simulink model "PIL_NO_RPI"  (R2021a)
settings: Solver=FixedStepAuto  StartTime=0.0  StopTime=50  FixedStep=0.001  RelTol=1e-3  EnableMultiTasking=on
undefined symbols (not defined in the file or in its folder): act_dmp, act_omega, Actuator, Aerodynamics, aMode, Autopilot, c_b_WGS, c_be, c_flat, c_grav, c_h_geop0, c_h_geope, c_pa0, c_pe, c_r0, c_rot, c_rsma, c_Tmp0, d_siB_0, d_siB_max, d_siB_min, dd_siB_max, dd_siB_min, DiscIntNeverNeededParam, e_pa, e_Tmp, fin_maxrate, flag_I_act_switch, flag_I_aero_switch, flag_I_flat, flag_I_gravity_switch, flag_I_rot, hcr, HIL_Data, JMMM_0, JMMM_e, JSPB_e, lat_0, lon_0, Mass_Props, mB_0, mM_0, mM_e, p, pBII_0, phi, pMPB, pNPB, propellant_kg, prp_FBPB, prp_mdot, prp_T, psi, pSPB, q, qEG_0, qIB_0, qIE_0, r, sgc ... (+28)
libraries: simulink x46, simulink_extras x10, aerolibcommonsys x4
(part 17 of 21)

== system PIL_NO_RPI/Non-linear Flight Dynamic Model1/Subsystem1/GRM_Airframe/rb_eom/calc_bus_flight_dyn_bus_entries/q12_from_T12/q_R^3(R) ==
  DCM : Inport
  q_R^3(R) = TRUE : EnablePort
  (1-r11-r22+r33)^1/2 : Sqrt  SaturateOnIntegerOverflow=on
  Add : Sum  Inputs=+--+
  Constant : Constant
  Divide : Product  Inputs=*/
  Divide1 : Product  Inputs=*/
  Divide2 : Product  Inputs=*/
  Gain : Gain  Gain=0.5
  Saturation : Saturate  UpperLimit=inf  LowerLimit=eps
      settings: AttributesFormatString=|
      | %<UpperLimit>
      | %<LowerLimit>
  Subtract : Sum
  Subtract1 : Sum  Inputs=+-
  Subtract2 : Sum
  Vector Concatenate : Concatenate  NumInputs=4
  dcm11 : Selector  NumberOfDimensions=2  IndexMode=Zero-based  InputPortWidth=3  IndexOptions=Index vector (dialog),Index vector (dialog)  Indices=0,0  OutputSizes=1,1
  dcm12 : Selector  NumberOfDimensions=2  IndexMode=Zero-based  InputPortWidth=3  IndexOptions=Index vector (dialog),Index vector (dialog)  Indices=0,1  OutputSizes=1,1
  dcm13 : Selector  NumberOfDimensions=2  IndexMode=Zero-based  InputPortWidth=3  IndexOptions=Index vector (dialog),Index vector (dialog)  Indices=0,2  OutputSizes=1,1
  dcm21 : Selector  NumberOfDimensions=2  IndexMode=Zero-based  InputPortWidth=3  IndexOptions=Index vector (dialog),Index vector (dialog)  Indices=1,0  OutputSizes=1,1
  dcm22 : Selector  NumberOfDimensions=2  IndexMode=Zero-based  InputPortWidth=3  IndexOptions=Index vector (dialog),Index vector (dialog)  Indices=1,1  OutputSizes=1,1
  dcm23 : Selector  NumberOfDimensions=2  IndexMode=Zero-based  InputPortWidth=3  IndexOptions=Index vector (dialog),Index vector (dialog)  Indices=1,2  OutputSizes=1,1
  dcm31 : Selector  NumberOfDimensions=2  IndexMode=Zero-based  InputPortWidth=3  IndexOptions=Index vector (dialog),Index vector (dialog)  Indices=2,0  OutputSizes=1,1
  dcm32 : Selector  NumberOfDimensions=2  IndexMode=Zero-based  InputPortWidth=3  IndexOptions=Index vector (dialog),Index vector (dialog)  Indices=2,1  OutputSizes=1,1
  dcm33 : Selector  NumberOfDimensions=2  IndexMode=Zero-based  InputPortWidth=3  IndexOptions=Index vector (dialog),Index vector (dialog)  Indices=2,2  OutputSizes=1,1
  q_R^3(R) : Outport  VectorParamsAs1DForOutWhenUnconnected=off
  wires:
  Saturation/1 -> Divide1/2, Divide2/2, Vector Concatenate/3, Divide/2  "q3"
  Gain/1 -> q_R^3(R)/1
  Divide/1 -> Vector Concatenate/4  "q4"
  Vector Concatenate/1 -> Gain/1
  (1-r11-r22+r33)^1/2/1 -> Saturation/1
  Divide2/1 -> Vector Concatenate/2  "q2"
  Divide1/1 -> Vector Concatenate/1  "q1"
  Subtract/1 -> Divide2/1  "dcm23+dcm32"
  Subtract2/1 -> Divide1/1  "dcm31+dcm13"
  Subtract1/1 -> Divide/1  "dcm12-dcm21"
  dcm12/1 -> Subtract1/1  "dcm12"
  dcm21/1 -> Subtract1/2  "dcm21"
  dcm13/1 -> Subtract2/2  "dcm13"
  dcm31/1 -> Subtract2/1  "dcm31"
  dcm32/1 -> Subtract/2  "dcm32"
  dcm23/1 -> Subtract/1  "dcm23"
  Add/1 -> (1-r11-r22+r33)^1/2/1
  dcm33/1 -> Add/4  "dcm33"
  dcm22/1 -> Add/3  "dcm22"
  dcm11/1 -> Add/2  "dcm11"
  Constant/1 -> Add/1
  DCM/1 -> dcm13/1, dcm31/1, dcm23/1, dcm32/1, dcm11/1, dcm22/1, dcm33/1, dcm21/1, dcm12/1

== system PIL_NO_RPI/Non-linear Flight Dynamic Model1/Subsystem1/GRM_Airframe/rb_eom/eom_6dof/Rigid_Body_EOM_6_DOF/Integration ==
  d_pBII : Inport
  d_vBII : Inport  Port=2
  d_qIB : Inport  Port=3
  d_wBIB : Inport  Port=4
  x0 : Inport  Port=5
  Bus Creator : BusCreator  Inputs=6
  Reshape : Reshape  OutputDimensionality=Customize  OutputDimensions=[13,1]
  Reshape1 : Reshape  OutputDimensionality=Customize  OutputDimensions=[3,1]
  Reshape2 : Reshape  OutputDimensionality=Customize  OutputDimensions=[3,1]
  Selector : Selector  IndexMode=Zero-based  InputPortWidth=13  IndexOptions=Index vector (dialog)  Indices=0:2  OutputSizes=3
  Selector1 : Selector  IndexMode=Zero-based  InputPortWidth=13  IndexOptions=Index vector (dialog)  Indices=3:5  OutputSizes=3
  Selector2 : Selector  IndexMode=Zero-based  InputPortWidth=13  IndexOptions=Index vector (dialog)  Indices=6:9  OutputSizes=3
  Selector3 : Selector  IndexMode=Zero-based  InputPortWidth=13  IndexOptions=Index vector (dialog)  Indices=10:12  OutputSizes=3
  Vector Concatenate : Concatenate  NumInputs=4  ConcatenateDimension=2
  integration_eom : Integrator  InitialConditionSource=external
  normalize_quaternion : Subsystem
      mask help: normalize a quaternion
      mask Help:
      | Name:
      | 
      |     normalize_quaternion
      | 
      | Description:
      | 
      |     This block normalizes the quaternion q21. It should be used as a
      |     safety measure when computing quaternions.
      | 
      | Inputs  [size] [data type] [unit]:
      | 
      |     attitude quaternion q21  [4] [double] [-]
      | 
      | Outputs  [size] [data type] [unit]:
      | 
      |     normalized attitude quaternion q21  [4] [double] [-]
      mask Display: disp (' norm(q)')
  eom : Outport  VectorParamsAs1DForOutWhenUnconnected=off
  wires:
  normalize_quaternion/1(q_normalized) -> Bus Creator/3  "qIB"
  Reshape2/1 -> Bus Creator/6  "d_vBII"
  Reshape1/1 -> Bus Creator/5  "d_wBIB"
  Reshape/1 -> integration_eom/1  "d_x"
  d_pBII/1 -> Vector Concatenate/1
  d_vBII/1 -> Vector Concatenate/2, Reshape2/1
  d_qIB/1 -> Vector Concatenate/3
  d_wBIB/1 -> Vector Concatenate/4, Reshape1/1
  Vector Concatenate/1 -> Reshape/1  "d_x"
  integration_eom/1 -> Selector2/1, Selector3/1, Selector/1, Selector1/1  "x"
  x0/1 -> integration_eom/2
  Selector/1 -> Bus Creator/1  "pBII"
  Selector1/1 -> Bus Creator/2  "vBII"
  Selector2/1 -> normalize_quaternion/1(q)  "qIB"
  Selector3/1 -> Bus Creator/4  "wBIB"
  Bus Creator/1 -> eom/1  "eom_bus"

== system PIL_NO_RPI/Non-linear Flight Dynamic Model1/Subsystem1/GRM_Airframe/rb_eom/eom_6dof/Rigid_Body_EOM_6_DOF/T12_from_q12 ==
  note: Inputs [size]:
      |
      | quaternion q12 [4]
  note: Outputs [size]:
      |
      | direction cosine matrix T12 [3x3]
  q12 : Inport  PortDimensions=4
  Add : Sum  Inputs=+--+
  Add1 : Sum  Inputs=+-
  Add2 : Sum  Inputs=+-
  Add3 : Sum  Inputs=+-
  Add4 : Sum
  Add5 : Sum
  Add6 : Sum  Inputs=-+-+
  Add7 : Sum  Inputs=--++
  Add8 : Sum
  Demux : Demux
  Gain{1..12} (12 alike) : Gain  Gain=2
  Math Function{,1..11} (12 alike) : Math  Operator=square  SignedPower=on  SaturateOnIntegerOverflow=on
  Product{,1..11} (12 alike) : Product
  Vector Concatenate : Concatenate  NumInputs=3
  Vector Concatenate1 : Concatenate  NumInputs=3
  Vector Concatenate2 : Concatenate  NumInputs=3
  Vector Concatenate3 : Concatenate  NumInputs=3  Mode=Multidimensional array  ConcatenateDimension=2
  T12 : Outport  PortDimensions=[3 3]  VectorParamsAs1DForOutWhenUnconnected=off
  wires:
  Product10/1 -> Gain11/1
  Product11/1 -> Gain12/1
  Gain11/1 -> Add8/1
  Gain12/1 -> Add8/2
  Math Function8/1 -> Add7/1
  Math Function9/1 -> Add7/2
  Math Function11/1 -> Add7/4
  Math Function10/1 -> Add7/3
  Math Function4/1 -> Add6/1
  Math Function5/1 -> Add6/2
  Math Function7/1 -> Add6/4
  Math Function6/1 -> Add6/3
  Product8/1 -> Gain9/1
  Product9/1 -> Gain10/1
  Gain9/1 -> Add5/1
  Gain10/1 -> Add5/2
  Product6/1 -> Gain7/1
  Product7/1 -> Gain8/1
  Gain7/1 -> Add4/1
  Gain8/1 -> Add4/2
  Product4/1 -> Gain5/1
  Product5/1 -> Gain6/1
  Gain5/1 -> Add3/1
  Gain6/1 -> Add3/2
  Product2/1 -> Gain3/1
  Product3/1 -> Gain4/1
  Gain3/1 -> Add2/1
  Gain4/1 -> Add2/2
  Gain2/1 -> Add1/2
  Gain1/1 -> Add1/1
  Product1/1 -> Gain2/1
  Product/1 -> Gain1/1
  Math Function3/1 -> Add/4
  Math Function2/1 -> Add/3
  Math Function1/1 -> Add/2
  Math Function/1 -> Add/1
  Add7/1 -> Vector Concatenate2/3  "dcm33"
  Add8/1 -> Vector Concatenate2/2  "dcm23"
  Add3/1 -> Vector Concatenate2/1  "dcm13"
  Add2/1 -> Vector Concatenate1/3  "dcm32"
  Add6/1 -> Vector Concatenate1/2  "dcm22"
  Add4/1 -> Vector Concatenate1/1  "dcm12"
  Add5/1 -> Vector Concatenate/3  "dcm31"
  Add1/1 -> Vector Concatenate/2  "dcm21"
  Add/1 -> Vector Concatenate/1  "dcm11"
  Vector Concatenate1/1 -> Vector Concatenate3/2
  Vector Concatenate2/1 -> Vector Concatenate3/3
  Vector Concatenate/1 -> Vector Concatenate3/1
  Vector Concatenate3/1 -> T12/1
  Demux/4 -> Product3/2, Product11/2, Math Function11/1, Product5/2, Math Function3/1, Product1/2, Product9/2, Product7/2, Math Function7/1  "q4 / q0"
  Demux/3 -> Math Function2/1, Product1/1, Product8/2, Product7/1, Math Function6/1, Product10/2, Math Function10/1, Product4/2, Product2/2  "q3"
  Demux/2 -> Math Function1/1, Product/2, Product9/1, Product6/2, Math Function5/1, Math Function9/1, Product10/1, Product5/1, Product2/1  "q2"
  Demux/1 -> Product6/1, Math Function4/1, Math Function8/1, Product11/1, Product4/1, Product3/1, Math Function/1, Product/1, Product8/1  "q1"
  q12/1 -> Demux/1

== system PIL_NO_RPI/Non-linear Flight Dynamic Model1/Subsystem1/GRM_Airframe/rb_eom/eom_6dof/Rigid_Body_EOM_6_DOF/rb_eom_6dof ==
  note: d_wBIB = JBB \ (MBTB - d_JBB * wBIB - wBIB x (JBB*wBIB))
  FBTB : Inport
  mB : Inport  Port=2
  JBB : Inport  Port=3
  MBTB : Inport  Port=4
  d_JBB : Inport  Port=5
  qIB : Inport  Port=6
  vBII : Inport  Port=7
  wBIB : Inport  Port=8
  Divide : Product  Inputs=*/
  Divide1 : Product  Inputs=/*  Multiplication=Matrix(*)
  Product : Product  Multiplication=Matrix(*)
  Product1 : Product  Multiplication=Matrix(*)
  Saturation : Saturate  UpperLimit=Inf  LowerLimit=1e-6
      settings: AttributesFormatString=|
      | %<UpperLimit>
      | %<LowerLimit>
  Subtract : Sum  Inputs=+--
  calc_d_qIB : Subsystem
  cross_product : Subsystem
      mask help: cross product r3 = r1 x r2
      mask Help:
      | Name:
      | 
      |     cross_product
      | 
      | Description:
      | 
      |     This block implements the cross product r3 = r1 x r2.
      | 
      | Inputs  [size] [data type] [unit]:
      | 
      |     vector 1  [3] [double] [-]
      |     vector 2  [3] [double] [-]
      | 
      | Outputs  [size] [data type] [unit]:
      | 
      |     resulting vector  [3] [double] [-]
      mask Display: disp(' r3 = r1 x r2')
  r2_from_r1_trans_q21 : Subsystem
      mask help: transforms a vector from frame 1 to frame 2 by a quaternion
      mask Help:
      | Name:
      | 
      |     r2_from_r1_trans_q21
      | 
      | Description:
      | 
      |     This block implements the transformation of a vector from the frame 1
      |     to the frame 2 using the appropriate quaternion.
      | 
      | Inputs  [size] [data type] [unit]:
      | 
      |     vector in frame 1  [3] [double] [-]
      |     attitude quaternion q21  [4] [double] [-]
      | 
      | Outputs  [size] [data type] [unit]:
      | 
      |     vector in frame 2  [3] [double] [-]
      mask Display:
      | port_label('input', 1, 'r1')
      | port_label('input', 2, 'q21')
      | port_label('output', 1, 'r2')
      | disp('r_2 = q_{21} {\bf\cdot} r_1 {\bf\cdot} q_{21}^{\bf\prime}','texmode','on')
  d_pBII : Outport  VectorParamsAs1DForOutWhenUnconnected=off
  d_vBII : Outport  Port=2  VectorParamsAs1DForOutWhenUnconnected=off
  d_qIB : Outport  Port=3  VectorParamsAs1DForOutWhenUnconnected=off
  d_wBIB : Outport  Port=4  VectorParamsAs1DForOutWhenUnconnected=off
  wires:
  Saturation/1 -> Divide/2
  calc_d_qIB/1(d_qIB) -> d_qIB/1
  MBTB/1 -> Subtract/1
  Subtract/1 -> Divide1/2
  d_JBB/1 -> Product/1
  Product1/1 -> cross_product/2(r2)
  cross_product/1(r1_x_r2) -> Subtract/3
  Product/1 -> Subtract/2
  Divide1/1 -> d_wBIB/1
  wBIB/1 -> calc_d_qIB/2(wBIB), Product/2, cross_product/1(r1), Product1/2
  JBB/1 -> Divide1/1, Product1/1
  vBII/1 -> d_pBII/1
  r2_from_r1_trans_q21/1(r2) -> d_vBII/1  "aBII"
  qIB/1 -> calc_d_qIB/1(qIB), r2_from_r1_trans_q21/2(q21)
  Divide/1 -> r2_from_r1_trans_q21/1(r1)  "aBIB"
  mB/1 -> Saturation/1
  FBTB/1 -> Divide/1

== system PIL_NO_RPI/Non-linear Flight Dynamic Model1/Subsystem1/GRM_Airframe/stream_flow/calc_stream_flow/Subsystem1/AoA_Sideslip_Alphatot_Phi ==
  note: Inputs [size]
      |
      | vector vBEB [3]
  note: Outputs [size]
      |
      | bus [4]
      | 	al  [1]
      | 	be [1]
      | 	th  [1]
      | 	fi   [1]
  note: falls a_vBEB == 0
      | Alle Winkel = 0
  vBEB : Inport
  Bus Creator : BusCreator  Inputs=4
  Constant : Constant  Value=[1; 0; 0; 1]
  Demux : Demux
  Demux1 : Demux  Outputs=3
  Divide : Product  Inputs=*/
  Divide1 : Product  Inputs=*/
  Switch : Switch  Criteria=u2 ~= 0
  Trigonometric Function : Trigonometry  Operator=atan2
  Trigonometric Function1 : Trigonometry  Operator=asin
  Trigonometric Function2 : Trigonometry  Operator=acos
  Trigonometric Function3 : Trigonometry  Operator=atan2
  Vector Concatenate : Concatenate  NumInputs=4
  norm_of_vector : Subsystem
      mask help: computes the norm of a vector
      mask Help:
      | Name:
      | 
      |     norm_of_vector
      | 
      | Description:
      | 
      |     This block computes the L2-norm (length) of a vector.
      | 
      | Inputs  [size] [data type] [unit]:
      | 
      |     vector  [3] [double] [-]
      | 
      | Outputs  [size] [data type] [unit]:
      | 
      |     norm of vector  [1] [double] [-]
      mask Display: disp (' norm(r) ')
  aero_angles : Outport  VectorParamsAs1DForOutWhenUnconnected=off
  wires:
  Demux1/2 -> Vector Concatenate/2  "vBEB_y"
  Demux1/3 -> Vector Concatenate/3  "vBEB_z"
  Demux1/1 -> Vector Concatenate/1  "vBEB_x"
  Divide1/1 -> Trigonometric Function2/1
  Trigonometric Function3/1 -> Bus Creator/4  "fi"
  Trigonometric Function2/1 -> Bus Creator/3  "th"
  Demux/4 -> Divide1/2, Divide/2  "a_vBEB"
  Switch/1 -> Demux/1
  Vector Concatenate/1 -> Switch/1
  Constant/1 -> Switch/3
  Bus Creator/1 -> aero_angles/1  "aero_angles_bus"
  norm_of_vector/1(norm_of_vector) -> Vector Concatenate/4, Switch/2  "a_vBEB"
  Trigonometric Function1/1 -> Bus Creator/2  "be"
  vBEB/1 -> norm_of_vector/1(vector), Demux1/1
  Demux/3 -> Trigonometric Function/1, Trigonometric Function3/2  "vBEB_z"
  Trigonometric Function/1 -> Bus Creator/1  "al"
  Divide/1 -> Trigonometric Function1/1
  Demux/1 -> Divide1/1, Trigonometric Function/2  "vBEB_x"
  Demux/2 -> Trigonometric Function3/1, Divide/1  "vBEB_y"

== system PIL_NO_RPI/Non-linear Flight Dynamic Model1/Subsystem1/GRM_Airframe/stream_flow/calc_stream_flow/Subsystem1/calc_nondimensional_rates ==
  a_vB : Inport
  wBIB : Inport  Port=2
  Constant1 : Constant  Value=Aerodynamics.lref
      settings: AttributesFormatString=%<Value>
  Constant2 : Constant  Value=2
  Demux : Demux  Outputs=3
  Divide1 : Product  Inputs=/*/
  Product2 : Product
  Product3 : Product
  Product4 : Product
  Saturation1 : Saturate  UpperLimit=inf  LowerLimit=100*eps
      settings: AttributesFormatString=|
      | %<UpperLimit>
      | %<LowerLimit>
  Vector Concatenate : Concatenate  NumInputs=3
  wBIB_star : Outport  VectorParamsAs1DForOutWhenUnconnected=off
  wires:
  Demux/2 -> Product3/2
  Divide1/1 -> Product4/1, Product3/1, Product2/1
  Demux/3 -> Product4/2
  a_vB/1 -> Saturation1/1
  wBIB/1 -> Demux/1
  Product3/1 -> Vector Concatenate/2  "qBIB_star"
  Demux/1 -> Product2/2
  Saturation1/1 -> Divide1/1
  Constant1/1 -> Divide1/2
  Product4/1 -> Vector Concatenate/3  "rBIB_star"
  Product2/1 -> Vector Concatenate/1  "pBIB_star"
  Vector Concatenate/1 -> wBIB_star/1  "wBIB_star"
  Constant2/1 -> Divide1/3

== system PIL_NO_RPI/Non-linear Flight Dynamic Model1/Subsystem1/GRM_Airframe/stream_flow/calc_stream_flow/Subsystem1/norm_of_vector ==
  note: Outputs [size]:
      |
      | norm of vector [1]
  note: Inputs [size]:
      |
      | vector  [3]
  vector : Inport
  Dot Product1 : DotProduct  InputSameDT=on  OutDataTypeStr=Inherit: Inherit via internal rule
  Math Function1 : Math  Operator=sqrt  SignedPower=on  SaturateOnIntegerOverflow=on
  norm_of_vector : Outport  VectorParamsAs1DForOutWhenUnconnected=off
  wires:
  vector/1 -> Dot Product1/1, Dot Product1/2
  Math Function1/1 -> norm_of_vector/1
  Dot Product1/1 -> Math Function1/1

== system PIL_NO_RPI/Non-linear Flight Dynamic Model1/Subsystem1/GRM_Airframe/stream_flow/calc_stream_flow/velocity_vector_transformation/cross_product ==
  note: Outputs [size]:
      |
      | r1 x r2  [3x1]
  note: Inputs [size]:
      |
      | r1 [3x1]
      | r2 [3x1]
  r1 : Inport
  r2 : Inport  Port=2
  Demux2 : Demux  Outputs=[1;1;1]
      settings: DisplayOption=none
  Demux3 : Demux  Outputs=[1;1;1]
      settings: DisplayOption=none
  Product{2..7} (6 alike) : Product  InputSameDT=on  RndMeth=Zero  SaturateOnIntegerOverflow=on  OutDataTypeStr=Inherit: Same as first input
  Sum : Sum  Inputs=+-  InputSameDT=on  SaturateOnIntegerOverflow=on  OutDataTypeStr=Inherit: Same as first input
  Sum1 : Sum  Inputs=+-  InputSameDT=on  SaturateOnIntegerOverflow=on  OutDataTypeStr=Inherit: Same as first input
  Sum2 : Sum  Inputs=+-  InputSameDT=on  SaturateOnIntegerOverflow=on  OutDataTypeStr=Inherit: Same as first input
  Vector Concatenate : Concatenate  NumInputs=3  Mode=Multidimensional array
  r1_x_r2 : Outport  PortDimensions=[3,1]  VectorParamsAs1DForOutWhenUnconnected=off
  wires:
  Demux2/2 -> Product2/1, Product7/1
  Demux3/3 -> Product5/2, Product2/2
  Demux3/2 -> Product6/2, Product3/2
  Demux2/3 -> Product3/1, Product4/1
  Demux3/1 -> Product7/2, Product4/2
  Demux2/1 -> Product6/1, Product5/1
  Product2/1 -> Sum/1
  Product3/1 -> Sum/2
  Product4/1 -> Sum1/1
  Product5/1 -> Sum1/2
  Product6/1 -> Sum2/1
  Product7/1 -> Sum2/2
  Sum/1 -> Vector Concatenate/1
  Sum1/1 -> Vector Concatenate/2
  Sum2/1 -> Vector Concatenate/3
  r1/1 -> Demux2/1
  r2/1 -> Demux3/1
  Vector Concatenate/1 -> r1_x_r2/1

== system PIL_NO_RPI/Non-linear Flight Dynamic Model1/Subsystem1/GRM_Airframe/weight_and_balance/moi/moi_coordinate_transformation/3_rot_mat ==
  wi1 : Inport
  wi2 : Inport  Port=2
  wi3 : Inport  Port=3
  1. Rotation x-Achse : Subsystem
  1. Rotation y-Achse : Subsystem
  1. Rotation z-Achse : Subsystem
  2. Rotation x-Achse : Subsystem
  2. Rotation y-Achse : Subsystem
  2. Rotation z-Achse : Subsystem
  3. Rotation : Product  Inputs=***  Multiplication=Matrix(*)
  3. Rotation x-Achse : Subsystem
  3. Rotation y-Achse : Subsystem
  3. Rotation z-Achse : Subsystem
  Constant : Constant  Value=rot_1
  Constant1 : Constant  Value=rot_2
  Constant2 : Constant  Value=rot_3
  Multiport Switch : MultiPortSwitch
  Multiport Switch1 : MultiPortSwitch
  Multiport Switch2 : MultiPortSwitch
  T12 : Outport  VectorParamsAs1DForOutWhenUnconnected=off
  wires:
  Multiport Switch2/1 -> 3. Rotation/1
  Multiport Switch1/1 -> 3. Rotation/2
  Multiport Switch/1 -> 3. Rotation/3
  wi3/1 -> 3. Rotation x-Achse/1(alpha3), 3. Rotation z-Achse/1(alpha3), 3. Rotation y-Achse/1(alpha3)
  wi1/1 -> 1. Rotation z-Achse/1(alpha1), 1. Rotation y-Achse/1(alpha1), 1. Rotation x-Achse/1(alpha1)
  wi2/1 -> 2. Rotation z-Achse/1(alpha2), 2. Rotation y-Achse/1(alpha2), 2. Rotation x-Achse/1(alpha2)
  3. Rotation z-Achse/1(3Rot_Matrix_z) -> Multiport Switch2/4
  Constant/1 -> Multiport Switch/1
  1. Rotation x-Achse/1(1Rot_Matrix_x) -> Multiport Switch/2
  Constant1/1 -> Multiport Switch1/1
  1. Rotation y-Achse/1(1Rot_Matrix_y) -> Multiport Switch/3
  1. Rotation z-Achse/1(1Rot_Matrix_z) -> Multiport Switch/4
  Constant2/1 -> Multiport Switch2/1
  3. Rotation/1 -> T12/1  "T12"
  2. Rotation x-Achse/1(2Rot_Matrix_x) -> Multiport Switch1/2
  2. Rotation y-Achse/1(2Rot_Matrix_y) -> Multiport Switch1/3
  2. Rotation z-Achse/1(2Rot_Matrix_z) -> Multiport Switch1/4
  3. Rotation y-Achse/1(3Rot_Matrix_y) -> Multiport Switch2/3
  3. Rotation x-Achse/1(3Rot_Matrix_x) -> Multiport Switch2/2

== system PIL_NO_RPI/Non-linear Flight Dynamic Model1/Subsystem1/GRM_Airframe/weight_and_balance/moi/steiners_theorem_missile/create_deviation_matrix ==
  pBXB : Inport
  Add : Sum
  Add4 : Sum
  Add5 : Sum
  Demux : Demux  Outputs=3
  Gain : Gain  Gain=-1
  Gain1 : Gain  Gain=-1
  Gain3 : Gain  Gain=-1
  Product{1..6} (6 alike) : Product
  Vector Concatenate1 : Concatenate  NumInputs=3  Mode=Multidimensional array  ConcatenateDimension=2
  Vector Concatenate6 : Concatenate  NumInputs=3
  Vector Concatenate7 : Concatenate  NumInputs=3
  Vector Concatenate8 : Concatenate  NumInputs=3
  T_deviation : Outport  VectorParamsAs1DForOutWhenUnconnected=off
  wires:
  Add4/1 -> Vector Concatenate8/3
  Vector Concatenate6/1 -> Vector Concatenate1/1
  Vector Concatenate7/1 -> Vector Concatenate1/2
  Demux/1 -> Product3/1, Product4/1, Product5/2, Product5/1  "a"
  Demux/3 -> Product6/2, Product4/2, Product2/1, Product2/2  "c"
  Gain/1 -> Vector Concatenate7/1, Vector Concatenate6/2
  Gain3/1 -> Vector Concatenate8/2, Vector Concatenate7/3
  Vector Concatenate1/1 -> T_deviation/1
  Demux/2 -> Product3/2, Product1/2, Product1/1, Product6/1  "b"
  Add5/1 -> Vector Concatenate7/2
  Product6/1 -> Gain3/1
  Add/1 -> Vector Concatenate6/1
  Product1/1 -> Add5/1, Add/1
  Product5/1 -> Add4/2, Add5/2
  Product2/1 -> Add4/1, Add/2
  Gain1/1 -> Vector Concatenate8/1, Vector Concatenate6/3
  Product4/1 -> Gain1/1
  Product3/1 -> Gain/1
  Vector Concatenate8/1 -> Vector Concatenate1/3
  pBXB/1 -> Demux/1

== system PIL_NO_RPI/Non-linear Flight Dynamic Model1/Subsystem1/GRM_Airframe/weight_and_balance/moi/steiners_theorem_motor/create_deviation_matrix1 ==
  pBXB : Inport
  Add : Sum
  Add4 : Sum
  Add5 : Sum
  Demux : Demux  Outputs=3
  Gain : Gain  Gain=-1
  Gain1 : Gain  Gain=-1
  Gain3 : Gain  Gain=-1
  Product{1..6} (6 alike) : Product
  Vector Concatenate1 : Concatenate  NumInputs=3  Mode=Multidimensional array  ConcatenateDimension=2
  Vector Concatenate6 : Concatenate  NumInputs=3
  Vector Concatenate7 : Concatenate  NumInputs=3
  Vector Concatenate8 : Concatenate  NumInputs=3
  T_deviation : Outport  VectorParamsAs1DForOutWhenUnconnected=off
  wires:
  pBXB/1 -> Demux/1
  Vector Concatenate8/1 -> Vector Concatenate1/3
  Product3/1 -> Gain/1
  Product4/1 -> Gain1/1
  Gain1/1 -> Vector Concatenate6/3, Vector Concatenate8/1
  Product2/1 -> Add/2, Add4/1
  Product5/1 -> Add5/2, Add4/2
  Product1/1 -> Add/1, Add5/1
  Add/1 -> Vector Concatenate6/1
  Product6/1 -> Gain3/1
  Add5/1 -> Vector Concatenate7/2
  Demux/2 -> Product6/1, Product1/1, Product1/2, Product3/2  "b"
  Vector Concatenate1/1 -> T_deviation/1
  Gain3/1 -> Vector Concatenate7/3, Vector Concatenate8/2
  Gain/1 -> Vector Concatenate6/2, Vector Concatenate7/1
  Demux/3 -> Product2/2, Product2/1, Product4/2, Product6/2  "c"
  Demux/1 -> Product5/1, Product5/2, Product4/1, Product3/1  "a"
  Vector Concatenate7/1 -> Vector Concatenate1/2
  Vector Concatenate6/1 -> Vector Concatenate1/1
  Add4/1 -> Vector Concatenate8/3

== system PIL_NO_RPI/Non-linear Flight Dynamic Model2/GRM_Airframe/aerodynamics/aerodynamic_via_lookup/calc_aero_for_mom/launch_rail/initial_altitude ==
  Constant : Constant  Value=pBII_0
  Constant2 : Constant  Value=flag_I_flat
  Demux : Demux  Outputs=3
  Gain : Gain  Gain=-1
  Switch1 : Switch  Criteria=u2 > Threshold
  Terminator{,1..3} (4 alike) : Terminator
  trafo_E_to_geodetic : Subsystem  mask(Transformation der ECEF Position in geodätische Größen){}
      mask help: Dieser Block transformiert die Position im ECEF KOS in die geodätische Länge, Breite und Höhe
      mask init:
      | [c_mue, c_rsma, c_flat] = init_transformations_earth;
      mask Help:
      | Name:
      | 
      |     trafo_E_to_geodetic
      | 
      | Beschreibung:
      | 
      |     Dieser Block transformiert die Position im ECEF KOS in die geodätische
      |     Länge, Breite und Höhe.
      | 
      | Inputs   [size]  [data type] [unit]:
      | 
      |     pBEE    [3] [double] [m]
      | 
      | Outputs  [size]  [data type] [unit]:
      | 
      |     long  [1] [double] [rad]
      |     lat   [1] [double] [rad]
      |     alt   [1] [double] [m]
      | 
      | Parameter
      | 
      |    c_rsma
      |    c_flat
  hBE_0 : Outport  VectorParamsAs1DForOutWhenUnconnected=off
  wires:
  Switch1/1 -> hBE_0/1  "hBE_0"
  trafo_E_to_geodetic/1(lon) -> Terminator/1
  Constant/1 -> trafo_E_to_geodetic/1(pBEE), Demux/1
  trafo_E_to_geodetic/2(lat) -> Terminator1/1
  Demux/1 -> Terminator2/1
  Gain/1 -> Switch1/1
  Demux/3 -> Gain/1
  Demux/2 -> Terminator3/1
  trafo_E_to_geodetic/3(alt) -> Switch1/3  "hBE_0"
  Constant2/1 -> Switch1/2

== system PIL_NO_RPI/Non-linear Flight Dynamic Model2/GRM_Airframe/aerodynamics/aerodynamic_via_lookup/calc_aero_for_mom/launch_rail1/initial_altitude ==
  Constant : Constant  Value=pBII_0
  Constant2 : Constant  Value=flag_I_flat
  Demux : Demux  Outputs=3
  Gain : Gain  Gain=-1
  Switch1 : Switch  Criteria=u2 > Threshold
  Terminator{,1..3} (4 alike) : Terminator
  trafo_E_to_geodetic : Subsystem  mask(Transformation der ECEF Position in geodätische Größen){}
      mask help: Dieser Block transformiert die Position im ECEF KOS in die geodätische Länge, Breite und Höhe
      mask init:
      | [c_mue, c_rsma, c_flat] = init_transformations_earth;
      mask Help:
      | Name:
      | 
      |     trafo_E_to_geodetic
      | 
      | Beschreibung:
      | 
      |     Dieser Block transformiert die Position im ECEF KOS in die geodätische
      |     Länge, Breite und Höhe.
      | 
      | Inputs   [size]  [data type] [unit]:
      | 
      |     pBEE    [3] [double] [m]
      | 
      | Outputs  [size]  [data type] [unit]:
      | 
      |     long  [1] [double] [rad]
      |     lat   [1] [double] [rad]
      |     alt   [1] [double] [m]
      | 
      | Parameter
      | 
      |    c_rsma
      |    c_flat
  hBE_0 : Outport  VectorParamsAs1DForOutWhenUnconnected=off
  wires:
  Constant2/1 -> Switch1/2
  trafo_E_to_geodetic/3(alt) -> Switch1/3  "hBE_0"
  Demux/2 -> Terminator3/1
  Demux/3 -> Gain/1
  Gain/1 -> Switch1/1
  Demux/1 -> Terminator2/1
  trafo_E_to_geodetic/2(lat) -> Terminator1/1
  Constant/1 -> Demux/1, trafo_E_to_geodetic/1(pBEE)
  trafo_E_to_geodetic/1(lon) -> Terminator/1
  Switch1/1 -> hBE_0/1  "hBE_0"

== system PIL_NO_RPI/Non-linear Flight Dynamic Model2/GRM_Airframe/environment/WGS84_Gravitation/WGS84_2_ECEF/WGS84 Transformation Parameter /Subsystem ==
  b : Inport
  a : Inport  Port=2
  Add : Sum  Inputs=-+
  Add1 : Sum  Inputs=+-
  Divide : Product  Inputs=*/
  Divide1 : Product  Inputs=**
  Sqrt : Sqrt  SaturateOnIntegerOverflow=on
  a2 : Constant  Value=2
  e : Outport  VectorParamsAs1DForOutWhenUnconnected=off
  wires:
  Add/1 -> Divide/1
  Add1/1 -> Divide1/1
  Divide/1 -> Add1/2, Divide1/2  "f"
  Divide1/1 -> Sqrt/1
  a2/1 -> Add1/1
  b/1 -> Add/1
  a/1 -> Divide/2, Add/2
  Sqrt/1 -> e/1  "e"

== system PIL_NO_RPI/Non-linear Flight Dynamic Model2/GRM_Airframe/gravity/launch_rail/initial_altitude/trafo_E_to_geodetic/Geodetic_altitude ==
  pBEE : Inport
  c_rsma : Inport  Port=2
  c_flat : Inport  Port=3
  lat : Inport  Port=4
  Add : Sum
  Constant : Constant
  Gain : Gain  Gain=2
  Product : Product  Inputs=*/  InputSameDT=on  RndMeth=Zero  SaturateOnIntegerOverflow=on  OutDataTypeStr=Inherit: Same as first input
  Product1 : Product
  Product2 : Product
  Product3 : Product
  Product4 : Product  Inputs=*/  InputSameDT=on  RndMeth=Zero  SaturateOnIntegerOverflow=on  OutDataTypeStr=Inherit: Same as first input
  Product5 : Product  Inputs=3
  Selector : Selector  IndexMode=Zero-based  InputPortWidth=3  IndexOptions=Index vector (dialog)  Indices=0  OutputSizes=1
  Selector1 : Selector  IndexMode=Zero-based  InputPortWidth=3  IndexOptions=Index vector (dialog)  Indices=1  OutputSizes=1
  Sqrt : Sqrt  SaturateOnIntegerOverflow=on
  Sqrt1 : Sqrt  SaturateOnIntegerOverflow=on
  Subtract : Sum  Inputs=+-
  Subtract1 : Sum  Inputs=+-
  Sum : Sum  Inputs=+-  InputSameDT=on  SaturateOnIntegerOverflow=on  OutDataTypeStr=Inherit: Same as first input
  Trigonometric Function : Trigonometry
  cos(latGD) : Trigonometry  Operator=cos
  alt : Outport  VectorParamsAs1DForOutWhenUnconnected=off
  wires:
  lat/1 -> Trigonometric Function/1, cos(latGD)/1
  Sqrt/1 -> Product/1
  cos(latGD)/1 -> Product/2
  c_rsma/1 -> Product4/1
  Subtract/1 -> Product5/3
  Product/1 -> Sum/1
  Sum/1 -> alt/1  "alt"
  Selector/1 -> Product1/2, Product1/1
  Selector1/1 -> Product2/2, Product2/1
  Product1/1 -> Add/1
  Product2/1 -> Add/2
  Add/1 -> Sqrt/1
  pBEE/1 -> Selector1/1, Selector/1
  Product3/1 -> Subtract/2
  Gain/1 -> Subtract/1
  c_flat/1 -> Product3/1, Product3/2, Gain/1
  Sqrt1/1 -> Product4/2
  Subtract1/1 -> Sqrt1/1
  Constant/1 -> Subtract1/1
  Product5/1 -> Subtract1/2
  Trigonometric Function/1 -> Product5/2, Product5/1
  Product4/1 -> Sum/2

== system PIL_NO_RPI/Non-linear Flight Dynamic Model2/GRM_Airframe/gravity/launch_rail/initial_altitude/trafo_E_to_geodetic/Geodetic_latitude ==
  pBEE : Inport
  c_rsma : Inport  Port=2
  c_flat : Inport  Port=3
  Add : Sum
  Add1 : Sum
  Constant : Constant
  Demux1 : Demux  Outputs=[1;1;1]
      settings: DisplayOption=none
  Divide : Product  Inputs=*/
  Divide1 : Product  Inputs=*/
  Divide2 : Product  Inputs=*/
  Gain : Gain  Gain=2
  Product{,1..7} (8 alike) : Product
  Product{8..11} (4 alike) : Product  Inputs=3
  Sqrt : Sqrt  SaturateOnIntegerOverflow=on
  Subtract{,1..3} (4 alike) : Sum  Inputs=+-
  Trigonometric Function : Trigonometry  Operator=atan
  Trigonometric Function1 : Trigonometry  Operator=atan
  Trigonometric Function2 : Trigonometry
  Trigonometric Function3 : Trigonometry  Operator=cos
  lat : Outport  VectorParamsAs1DForOutWhenUnconnected=off
  wires:
  c_flat/1 -> [f]
  c_rsma/1 -> [a]
  pBEE/1 -> Demux1/1
  Demux1/3 -> [z]
  [a] -> Product/1
  [f] -> Subtract/2
  Demux1/1 -> Product1/2, Product1/1
  Demux1/2 -> Product2/2, Product2/1
  [a] -> Product4/2, Product4/1
  [b] -> Product5/2, Product5/1
  [f] -> Product3/2, Product3/1, Gain/1
  [z] -> Product6/1
  [a] -> Product6/2
  Trigonometric Function/1 -> Trigonometric Function3/1, Trigonometric Function2/1
  [P] -> Product7/1
  [b] -> Product7/2
  [z] -> Add1/1
  [b] -> Product10/2
  [P] -> Subtract3/1
  Subtract1/1 -> Product11/1
  [a] -> Product11/2
  Trigonometric Function1/1 -> lat/1  "lat"
  Constant/1 -> Subtract/1
  Subtract/1 -> Product/2
  Product/1 -> [b]
  Product1/1 -> Add/1
  Product2/1 -> Add/2
  Add/1 -> Sqrt/1
  Sqrt/1 -> [P]
  Product3/1 -> Subtract1/2
  Gain/1 -> Subtract1/1
  Product4/1 -> Subtract2/1
  Product5/1 -> Subtract2/2, Divide/2
  Subtract2/1 -> Divide/1
  Product6/1 -> Divide1/1
  Product7/1 -> Divide1/2
  Divide1/1 -> Trigonometric Function/1
  Divide2/1 -> Trigonometric Function1/1
  Trigonometric Function2/1 -> Product8/2, Product8/3, Product8/1
  Trigonometric Function3/1 -> Product9/2, Product9/3, Product9/1
  Product8/1 -> Product10/3
  Product10/1 -> Add1/2
  Add1/1 -> Divide2/1
  Subtract3/1 -> Divide2/2
  Product11/1 -> Subtract3/2
  Product9/1 -> Product11/3
  Divide/1 -> Product10/1

== system PIL_NO_RPI/Non-linear Flight Dynamic Model2/GRM_Airframe/motion_kinematics/calc_motion_kinematics/calc_transformation_matrix/q31_from_q32_mul_q1/normalize_quaternion ==
  note: Inputs [size]:
      |
      | q [4]
  note: Outputs [size]:
      |
      | q_norm [4]
  q : Inport
  Add : Sum  Inputs=++++
  Demux : Demux  Outputs=[1;1;1;1]
  Math Function : Math  Operator=sqrt  SignedPower=on  SaturateOnIntegerOverflow=on
  Product : Product  Inputs=*/  InputSameDT=on  RndMeth=Zero  SaturateOnIntegerOverflow=on  OutDataTypeStr=Inherit: Same as first input
  Product{1..4} (4 alike) : Product  RndMeth=Zero
  q_normalized : Outport  VectorParamsAs1DForOutWhenUnconnected=off
  wires:
  Product/1 -> q_normalized/1
  q/1 -> Product/1, Demux/1
  Demux/1 -> Product1/1, Product1/2
  Demux/2 -> Product2/1, Product2/2
  Demux/3 -> Product3/1, Product3/2
  Demux/4 -> Product4/1, Product4/2
  Product4/1 -> Add/4
  Product3/1 -> Add/3
  Product2/1 -> Add/2
  Product1/1 -> Add/1
  Add/1 -> Math Function/1
  Math Function/1 -> Product/2

== system PIL_NO_RPI/Non-linear Flight Dynamic Model2/GRM_Airframe/motion_kinematics/calc_motion_kinematics/calc_transformation_matrix/q31_from_q32_mul_q2/normalize_quaternion ==
  note: Inputs [size]:
      |
      | q [4]
  note: Outputs [size]:
      |
      | q_norm [4]
  q : Inport
  Add : Sum  Inputs=++++
  Demux : Demux  Outputs=[1;1;1;1]
  Math Function : Math  Operator=sqrt  SignedPower=on  SaturateOnIntegerOverflow=on
  Product : Product  Inputs=*/  InputSameDT=on  RndMeth=Zero  SaturateOnIntegerOverflow=on  OutDataTypeStr=Inherit: Same as first input
  Product{1..4} (4 alike) : Product  RndMeth=Zero
  q_normalized : Outport  VectorParamsAs1DForOutWhenUnconnected=off
  wires:
  Product/1 -> q_normalized/1
  q/1 -> Product/1, Demux/1
  Demux/1 -> Product1/1, Product1/2
  Demux/2 -> Product2/1, Product2/2
  Demux/3 -> Product3/1, Product3/2
  Demux/4 -> Product4/1, Product4/2
  Product4/1 -> Add/4
  Product3/1 -> Add/3
  Product2/1 -> Add/2
  Product1/1 -> Add/1
  Add/1 -> Math Function/1
  Math Function/1 -> Product/2

== system PIL_NO_RPI/Non-linear Flight Dynamic Model2/GRM_Airframe/motion_kinematics/calc_motion_kinematics/calc_transformation_matrix/q31_from_q32_mul_q21/normalize_quaternion ==
  note: Inputs [size]:
      |
      | q [4]
  note: Outputs [size]:
      |
      | q_norm [4]
  q : Inport
  Add : Sum  Inputs=++++
  Demux : Demux  Outputs=[1;1;1;1]
  Math Function : Math  Operator=sqrt  SignedPower=on  SaturateOnIntegerOverflow=on
  Product : Product  Inputs=*/  InputSameDT=on  RndMeth=Zero  SaturateOnIntegerOverflow=on  OutDataTypeStr=Inherit: Same as first input
  Product{1..4} (4 alike) : Product  RndMeth=Zero
  q_normalized : Outport  VectorParamsAs1DForOutWhenUnconnected=off
  wires:
  Product/1 -> q_normalized/1
  q/1 -> Product/1, Demux/1
  Demux/1 -> Product1/1, Product1/2
  Demux/2 -> Product2/1, Product2/2
  Demux/3 -> Product3/1, Product3/2
  Demux/4 -> Product4/1, Product4/2
  Product4/1 -> Add/4
  Product3/1 -> Add/3
  Product2/1 -> Add/2
  Product1/1 -> Add/1
  Add/1 -> Math Function/1
  Math Function/1 -> Product/2

== system PIL_NO_RPI/Non-linear Flight Dynamic Model2/GRM_Airframe/motion_kinematics/calc_motion_kinematics/earth_rotation/quaternion_integration/Subsystem1 ==
  wEIE : Inport
  qIE : Inport  Port=2
  Add : Sum  Inputs=4
  Constant8 : Constant  Value=0
  Demux : Demux
  Demux1 : Demux  Outputs=3
  Gain : Gain  Gain=0.5
  Product{1..4} (4 alike) : Product
  Product5 : Product  Multiplication=Matrix(*)
  Q_1 : Constant  Value=[0 0 0 1; 0 0 1 0; 0 -1 0 0; -1 0 0 0]
  Q_2 : Constant  Value=[0 0 -1 0; 0 0 0 1; 1 0 0 0; 0 -1 0 0]
  Q_3 : Constant  Value=[0 1 0 0; -1 0 0 0; 0 0 0 1; 0 0 -1 0]
  Q_4 : Constant  Value=[1 0 0 0; 0 1 0 0; 0 0 1 0; 0 0 0 1]
  Vector Concatenate : Concatenate  NumInputs=4
  conjugate_quaternion1 : Subsystem
      mask help: conjugate a quaternion
      mask Help:
      | Name:
      | 
      |     conjugate_quaternion
      | 
      | Description:
      | 
      |     computes the conjugate quaternion
      | 
      | Inputs  [size] [data type] [unit]:
      | 
      |     quaternion q_2_1  [4] [double] [-]
      | 
      | Outputs  [size] [data type] [unit]:
      | 
      |     conjugated quaternion q_1_2  [4] [double] [-]
      mask Display: disp (' conj(q)')
  conjugate_quaternion2 : Subsystem
      mask help: conjugate a quaternion
      mask Help:
      | Name:
      | 
      |     conjugate_quaternion
      | 
      | Description:
      | 
      |     computes the conjugate quaternion
      | 
      | Inputs  [size] [data type] [unit]:
      | 
      |     quaternion q_2_1  [4] [double] [-]
      | 
      | Outputs  [size] [data type] [unit]:
      | 
      |     conjugated quaternion q_1_2  [4] [double] [-]
      mask Display: disp (' conj(q)')
  d_qIE : Outport  VectorParamsAs1DForOutWhenUnconnected=off
  wires:
  conjugate_quaternion2/1(q_conj) -> d_qIE/1  "d_qIE"
  wEIE/1 -> Demux1/1
  Demux/2 -> Product2/2  "w2"
  conjugate_quaternion1/1(q_conj) -> Product5/2  "qEI"
  Demux1/2 -> Vector Concatenate/2
  Demux/3 -> Product3/2  "w3"
  Q_4/1 -> Product4/1
  Product1/1 -> Add/1
  Gain/1 -> conjugate_quaternion2/1(q)  "d_qEI"
  Product5/1 -> Gain/1
  Q_2/1 -> Product2/1
  Vector Concatenate/1 -> Demux/1
  Demux/1 -> Product1/2  "w1"
  Demux1/1 -> Vector Concatenate/1
  Constant8/1 -> Vector Concatenate/4
  Q_1/1 -> Product1/1
  Q_3/1 -> Product3/1
  Product3/1 -> Add/3
  Product4/1 -> Add/4
  Demux/4 -> Product4/2  "w4"
  Add/1 -> Product5/1
  Product2/1 -> Add/2
  Demux1/3 -> Vector Concatenate/3
  qIE/1 -> conjugate_quaternion1/1(q)

== system PIL_NO_RPI/Non-linear Flight Dynamic Model2/GRM_Airframe/motion_kinematics/calc_motion_kinematics/earth_rotation/quaternion_integration/T12_from_q12 ==
  note: Outputs [size]:
      |
      | direction cosine matrix T12 [3x3]
  note: Inputs [size]:
      |
      | quaternion q12 [4]
  q12 : Inport  PortDimensions=4
  Add : Sum  Inputs=+--+
  Add1 : Sum  Inputs=+-
  Add2 : Sum  Inputs=+-
  Add3 : Sum  Inputs=+-
  Add4 : Sum
  Add5 : Sum
  Add6 : Sum  Inputs=-+-+
  Add7 : Sum  Inputs=--++
  Add8 : Sum
  Demux : Demux
  Gain{1..12} (12 alike) : Gain  Gain=2
  Math Function{,1..11} (12 alike) : Math  Operator=square  SignedPower=on  SaturateOnIntegerOverflow=on
  Product{,1..11} (12 alike) : Product
  Vector Concatenate : Concatenate  NumInputs=3
  Vector Concatenate1 : Concatenate  NumInputs=3
  Vector Concatenate2 : Concatenate  NumInputs=3
  Vector Concatenate3 : Concatenate  NumInputs=3  Mode=Multidimensional array  ConcatenateDimension=2
  T12 : Outport  PortDimensions=[3 3]  VectorParamsAs1DForOutWhenUnconnected=off
  wires:
  q12/1 -> Demux/1
  Demux/1 -> Product8/1, Product/1, Math Function/1, Product3/1, Product4/1, Product11/1, Math Function8/1, Math Function4/1, Product6/1  "q1"
  Demux/2 -> Product2/1, Product5/1, Product10/1, Math Function9/1, Math Function5/1, Product6/2, Product9/1, Product/2, Math Function1/1  "q2"
  Demux/3 -> Product2/2, Product4/2, Math Function10/1, Product10/2, Math Function6/1, Product7/1, Product8/2, Product1/1, Math Function2/1  "q3"
  Demux/4 -> Math Function7/1, Product7/2, Product9/2, Product1/2, Math Function3/1, Product5/2, Math Function11/1, Product11/2, Product3/2  "q4 / q0"
  Vector Concatenate3/1 -> T12/1
  Vector Concatenate/1 -> Vector Concatenate3/1
  Vector Concatenate2/1 -> Vector Concatenate3/3
  Vector Concatenate1/1 -> Vector Concatenate3/2
  Add/1 -> Vector Concatenate/1  "dcm11"
  Add1/1 -> Vector Concatenate/2  "dcm21"
  Add5/1 -> Vector Concatenate/3  "dcm31"
  Add4/1 -> Vector Concatenate1/1  "dcm12"
  Add6/1 -> Vector Concatenate1/2  "dcm22"
  Add2/1 -> Vector Concatenate1/3  "dcm32"
  Add3/1 -> Vector Concatenate2/1  "dcm13"
  Add8/1 -> Vector Concatenate2/2  "dcm23"
  Add7/1 -> Vector Concatenate2/3  "dcm33"
  Math Function/1 -> Add/1
  Math Function1/1 -> Add/2
  Math Function2/1 -> Add/3
  Math Function3/1 -> Add/4
  Product/1 -> Gain1/1
  Product1/1 -> Gain2/1
  Gain1/1 -> Add1/1
  Gain2/1 -> Add1/2
  Gain4/1 -> Add2/2
  Gain3/1 -> Add2/1
  Product3/1 -> Gain4/1
  Product2/1 -> Gain3/1
  Gain6/1 -> Add3/2
  Gain5/1 -> Add3/1
  Product5/1 -> Gain6/1
  Product4/1 -> Gain5/1
  Gain8/1 -> Add4/2
  Gain7/1 -> Add4/1
  Product7/1 -> Gain8/1
  Product6/1 -> Gain7/1
  Gain10/1 -> Add5/2
  Gain9/1 -> Add5/1
  Product9/1 -> Gain10/1
  Product8/1 -> Gain9/1
  Math Function6/1 -> Add6/3
  Math Function7/1 -> Add6/4
  Math Function5/1 -> Add6/2
  Math Function4/1 -> Add6/1
  Math Function10/1 -> Add7/3
  Math Function11/1 -> Add7/4
  Math Function9/1 -> Add7/2
  Math Function8/1 -> Add7/1
  Gain12/1 -> Add8/2
  Gain11/1 -> Add8/1
  Product11/1 -> Gain12/1
  Product10/1 -> Gain11/1

== system PIL_NO_RPI/Non-linear Flight Dynamic Model2/GRM_Airframe/motion_kinematics/calc_motion_kinematics/earth_rotation/quaternion_integration1/Subsystem1 ==
  wGEG : Inport
  qEG : Inport  Port=2
  Add : Sum  Inputs=4
  Constant8 : Constant  Value=0
  Demux : Demux
  Demux1 : Demux  Outputs=3
  Gain : Gain  Gain=0.5
  Product{1..4} (4 alike) : Product
  Product5 : Product  Multiplication=Matrix(*)
  Q_1 : Constant  Value=[0 0 0 1; 0 0 1 0; 0 -1 0 0; -1 0 0 0]
  Q_2 : Constant  Value=[0 0 -1 0; 0 0 0 1; 1 0 0 0; 0 -1 0 0]
  Q_3 : Constant  Value=[0 1 0 0; -1 0 0 0; 0 0 0 1; 0 0 -1 0]
  Q_4 : Constant  Value=[1 0 0 0; 0 1 0 0; 0 0 1 0; 0 0 0 1]
  Vector Concatenate : Concatenate  NumInputs=4
  conjugate_quaternion1 : Subsystem
      mask help: conjugate a quaternion
      mask Help:
      | Name:
      | 
      |     conjugate_quaternion
      | 
      | Description:
      | 
      |     computes the conjugate quaternion
      | 
      | Inputs  [size] [data type] [unit]:
      | 
      |     quaternion q_2_1  [4] [double] [-]
      | 
      | Outputs  [size] [data type] [unit]:
      | 
      |     conjugated quaternion q_1_2  [4] [double] [-]
      mask Display: disp (' conj(q)')
  conjugate_quaternion2 : Subsystem
      mask help: conjugate a quaternion
      mask Help:
      | Name:
      | 
      |     conjugate_quaternion
      | 
      | Description:
      | 
      |     computes the conjugate quaternion
      | 
      | Inputs  [size] [data type] [unit]:
      | 
      |     quaternion q_2_1  [4] [double] [-]
      | 
      | Outputs  [size] [data type] [unit]:
      | 
      |     conjugated quaternion q_1_2  [4] [double] [-]
      mask Display: disp (' conj(q)')
  d_qEG : Outport  VectorParamsAs1DForOutWhenUnconnected=off
  wires:
  qEG/1 -> conjugate_quaternion1/1(q)
  Demux1/3 -> Vector Concatenate/3
  Product2/1 -> Add/2
  Add/1 -> Product5/1
  Demux/4 -> Product4/2  "w4"
  Product4/1 -> Add/4
  Product3/1 -> Add/3
  Q_3/1 -> Product3/1
  Q_1/1 -> Product1/1
  Constant8/1 -> Vector Concatenate/4
  Demux1/1 -> Vector Concatenate/1
  Demux/1 -> Product1/2  "w1"
  Vector Concatenate/1 -> Demux/1
  Q_2/1 -> Product2/1
  Product5/1 -> Gain/1
  Gain/1 -> conjugate_quaternion2/1(q)  "d_qGE"
  Product1/1 -> Add/1
  Q_4/1 -> Product4/1
  Demux/3 -> Product3/2  "w3"
  Demux1/2 -> Vector Concatenate/2
  conjugate_quaternion1/1(q_conj) -> Product5/2  "qGE"
  Demux/2 -> Product2/2  "w2"
  wGEG/1 -> Demux1/1
  conjugate_quaternion2/1(q_conj) -> d_qEG/1  "d_qEG"

== system PIL_NO_RPI/Non-linear Flight Dynamic Model2/GRM_Airframe/motion_kinematics/calc_motion_kinematics/earth_rotation/quaternion_integration1/T12_from_q12 ==
  note: Outputs [size]:
      |
      | direction cosine matrix T12 [3x3]
  note: Inputs [size]:
      |
      | quaternion q12 [4]
  q12 : Inport  PortDimensions=4
  Add : Sum  Inputs=+--+
  Add1 : Sum  Inputs=+-
  Add2 : Sum  Inputs=+-
  Add3 : Sum  Inputs=+-
  Add4 : Sum
  Add5 : Sum
  Add6 : Sum  Inputs=-+-+
  Add7 : Sum  Inputs=--++
  Add8 : Sum
  Demux : Demux
  Gain{1..12} (12 alike) : Gain  Gain=2
  Math Function{,1..11} (12 alike) : Math  Operator=square  SignedPower=on  SaturateOnIntegerOverflow=on
  Product{,1..11} (12 alike) : Product
  Vector Concatenate : Concatenate  NumInputs=3
  Vector Concatenate1 : Concatenate  NumInputs=3
  Vector Concatenate2 : Concatenate  NumInputs=3
  Vector Concatenate3 : Concatenate  NumInputs=3  Mode=Multidimensional array  ConcatenateDimension=2
  T12 : Outport  PortDimensions=[3 3]  VectorParamsAs1DForOutWhenUnconnected=off
  wires:
  q12/1 -> Demux/1
  Demux/1 -> Product8/1, Product/1, Math Function/1, Product3/1, Product4/1, Product11/1, Math Function8/1, Math Function4/1, Product6/1  "q1"
  Demux/2 -> Product2/1, Product5/1, Product10/1, Math Function9/1, Math Function5/1, Product6/2, Product9/1, Product/2, Math Function1/1  "q2"
  Demux/3 -> Product2/2, Product4/2, Math Function10/1, Product10/2, Math Function6/1, Product7/1, Product8/2, Product1/1, Math Function2/1  "q3"
  Demux/4 -> Math Function7/1, Product7/2, Product9/2, Product1/2, Math Function3/1, Product5/2, Math Function11/1, Product11/2, Product3/2  "q4 / q0"
  Vector Concatenate3/1 -> T12/1
  Vector Concatenate/1 -> Vector Concatenate3/1
  Vector Concatenate2/1 -> Vector Concatenate3/3
  Vector Concatenate1/1 -> Vector Concatenate3/2
  Add/1 -> Vector Concatenate/1  "dcm11"
  Add1/1 -> Vector Concatenate/2  "dcm21"
  Add5/1 -> Vector Concatenate/3  "dcm31"
  Add4/1 -> Vector Concatenate1/1  "dcm12"
  Add6/1 -> Vector Concatenate1/2  "dcm22"
  Add2/1 -> Vector Concatenate1/3  "dcm32"
  Add3/1 -> Vector Concatenate2/1  "dcm13"
  Add8/1 -> Vector Concatenate2/2  "dcm23"
  Add7/1 -> Vector Concatenate2/3  "dcm33"
  Math Function/1 -> Add/1
  Math Function1/1 -> Add/2
  Math Function2/1 -> Add/3
  Math Function3/1 -> Add/4
  Product/1 -> Gain1/1
  Product1/1 -> Gain2/1
  Gain1/1 -> Add1/1
  Gain2/1 -> Add1/2
  Gain4/1 -> Add2/2
  Gain3/1 -> Add2/1
  Product3/1 -> Gain4/1
  Product2/1 -> Gain3/1
  Gain6/1 -> Add3/2
  Gain5/1 -> Add3/1
  Product5/1 -> Gain6/1
  Product4/1 -> Gain5/1
  Gain8/1 -> Add4/2
  Gain7/1 -> Add4/1
  Product7/1 -> Gain8/1
  Product6/1 -> Gain7/1
  Gain10/1 -> Add5/2
  Gain9/1 -> Add5/1
  Product9/1 -> Gain10/1
  Product8/1 -> Gain9/1
  Math Function6/1 -> Add6/3
  Math Function7/1 -> Add6/4
  Math Function5/1 -> Add6/2
  Math Function4/1 -> Add6/1
  Math Function10/1 -> Add7/3
  Math Function11/1 -> Add7/4
  Math Function9/1 -> Add7/2
  Math Function8/1 -> Add7/1
  Gain12/1 -> Add8/2
  Gain11/1 -> Add8/1
  Product11/1 -> Gain12/1
  Product10/1 -> Gain11/1

== system PIL_NO_RPI/Non-linear Flight Dynamic Model2/GRM_Airframe/rb_eom/calc_bus_flight_dyn_bus_entries/Subsystem2/trafo_E_to_geodetic/Geodetic_altitude ==
  pBEE : Inport
  c_rsma : Inport  Port=2
  c_flat : Inport  Port=3
  lat : Inport  Port=4
  Add : Sum
  Constant : Constant
  Gain : Gain  Gain=2
  Product : Product  Inputs=*/  InputSameDT=on  RndMeth=Zero  SaturateOnIntegerOverflow=on  OutDataTypeStr=Inherit: Same as first input
  Product1 : Product
  Product2 : Product
  Product3 : Product
  Product4 : Product  Inputs=*/  InputSameDT=on  RndMeth=Zero  SaturateOnIntegerOverflow=on  OutDataTypeStr=Inherit: Same as first input
  Product5 : Product  Inputs=3
  Selector : Selector  IndexMode=Zero-based  InputPortWidth=3  IndexOptions=Index vector (dialog)  Indices=0  OutputSizes=1
  Selector1 : Selector  IndexMode=Zero-based  InputPortWidth=3  IndexOptions=Index vector (dialog)  Indices=1  OutputSizes=1
  Sqrt : Sqrt  SaturateOnIntegerOverflow=on
  Sqrt1 : Sqrt  SaturateOnIntegerOverflow=on
  Subtract : Sum  Inputs=+-
  Subtract1 : Sum  Inputs=+-
  Sum : Sum  Inputs=+-  InputSameDT=on  SaturateOnIntegerOverflow=on  OutDataTypeStr=Inherit: Same as first input
  Trigonometric Function : Trigonometry
  cos(latGD) : Trigonometry  Operator=cos
  alt : Outport  VectorParamsAs1DForOutWhenUnconnected=off
  wires:
  lat/1 -> Trigonometric Function/1, cos(latGD)/1
  Sqrt/1 -> Product/1
  cos(latGD)/1 -> Product/2
  c_rsma/1 -> Product4/1
  Subtract/1 -> Product5/3
  Product/1 -> Sum/1
  Sum/1 -> alt/1  "alt"
  Selector/1 -> Product1/2, Product1/1
  Selector1/1 -> Product2/2, Product2/1
  Product1/1 -> Add/1
  Product2/1 -> Add/2
  Add/1 -> Sqrt/1
  pBEE/1 -> Selector1/1, Selector/1
  Product3/1 -> Subtract/2
  Gain/1 -> Subtract/1
  c_flat/1 -> Product3/1, Product3/2, Gain/1
  Sqrt1/1 -> Product4/2
  Subtract1/1 -> Sqrt1/1
  Constant/1 -> Subtract1/1
  Product5/1 -> Subtract1/2
  Trigonometric Function/1 -> Product5/2, Product5/1
  Product4/1 -> Sum/2

== system PIL_NO_RPI/Non-linear Flight Dynamic Model2/GRM_Airframe/rb_eom/calc_bus_flight_dyn_bus_entries/Subsystem2/trafo_E_to_geodetic/Geodetic_latitude ==
  pBEE : Inport
  c_rsma : Inport  Port=2
  c_flat : Inport  Port=3
  Add : Sum
  Add1 : Sum
  Constant : Constant
  Demux1 : Demux  Outputs=[1;1;1]
      settings: DisplayOption=none
  Divide : Product  Inputs=*/
  Divide1 : Product  Inputs=*/
  Divide2 : Product  Inputs=*/
  Gain : Gain  Gain=2
  Product{,1..7} (8 alike) : Product
  Product{8..11} (4 alike) : Product  Inputs=3
  Sqrt : Sqrt  SaturateOnIntegerOverflow=on
  Subtract{,1..3} (4 alike) : Sum  Inputs=+-
  Trigonometric Function : Trigonometry  Operator=atan
  Trigonometric Function1 : Trigonometry  Operator=atan
  Trigonometric Function2 : Trigonometry
  Trigonometric Function3 : Trigonometry  Operator=cos
  lat : Outport  VectorParamsAs1DForOutWhenUnconnected=off
  wires:
  c_flat/1 -> [f]
  c_rsma/1 -> [a]
  pBEE/1 -> Demux1/1
  Demux1/3 -> [z]
  [a] -> Product/1
  [f] -> Subtract/2
  Demux1/1 -> Product1/2, Product1/1
  Demux1/2 -> Product2/2, Product2/1
  [a] -> Product4/2, Product4/1
  [b] -> Product5/2, Product5/1
  [f] -> Product3/2, Product3/1, Gain/1
  [z] -> Product6/1
  [a] -> Product6/2
  Trigonometric Function/1 -> Trigonometric Function3/1, Trigonometric Function2/1
  [P] -> Product7/1
  [b] -> Product7/2
  [z] -> Add1/1
  [b] -> Product10/2
  [P] -> Subtract3/1
  Subtract1/1 -> Product11/1
  [a] -> Product11/2
  Trigonometric Function1/1 -> lat/1  "lat"
  Constant/1 -> Subtract/1
  Subtract/1 -> Product/2
  Product/1 -> [b]
  Product1/1 -> Add/1
  Product2/1 -> Add/2
  Add/1 -> Sqrt/1
  Sqrt/1 -> [P]
  Product3/1 -> Subtract1/2
  Gain/1 -> Subtract1/1
  Product4/1 -> Subtract2/1
  Product5/1 -> Subtract2/2, Divide/2
  Subtract2/1 -> Divide/1
  Product6/1 -> Divide1/1
  Product7/1 -> Divide1/2
  Divide1/1 -> Trigonometric Function/1
  Divide2/1 -> Trigonometric Function1/1
  Trigonometric Function2/1 -> Product8/2, Product8/3, Product8/1
  Trigonometric Function3/1 -> Product9/2, Product9/3, Product9/1
  Product8/1 -> Product10/3
  Product10/1 -> Add1/2
  Add1/1 -> Divide2/1
  Subtract3/1 -> Divide2/2
  Product11/1 -> Subtract3/2
  Product9/1 -> Product11/3
  Divide/1 -> Product10/1
